simulink model "quad_new_leg_raibert_strategy_v5"  (R2022b)
settings: Solver=ode15s  StartTime=0.0  StopTime=5  RelTol=1e-3
undefined symbols (not defined in the file or in its folder): body, ctrl, ground, planner, X, Y, Z
libraries: nesl_utility x73, sm_lib x42, slpidlib x24, simulink x5, Contact_Forces_Lib x4, Parts_Lib x4, fl_lib x1, sharedtransform x1, dspstat3 x1
(part 5 of 5)

== system quad_new_leg_raibert_strategy_v5/leg_rr/u_joint_ctrl  ==
  tgt_angle : Inport
  has_ctrl : Inport  Port=2
  PID Controller : slpidlib/PID Controller  Controller=PID  Form=Parallel  TimeDomain=Continuous-time  UseExternalTs=off  SampleTime=-1  IntegratorMethod=Forward Euler  FilterMethod=Forward Euler  ControllerParametersSource=internal  P=ctrl.pos_kp  I=ctrl.pos_ki  UseKiTs=off  D=ctrl.pos_kd  N=100  UseFilter=on  TunerSelectOption=Transfer Function Based (PID Tuner App)  InitialConditionSource=internal  InitialConditionForIntegrator=0  InitialConditionForFilter=0  DifferentiatorICPrevScaledInput=0  ExternalReset=none  TrackingMode=off  Kt=1  LimitOutput=off  SatLimitsSource=internal  UpperSaturationLimit=inf  LowerSaturationLimit=-inf  LinearizeAsGain=on  AntiWindupMode=none  Kb=1  LimitIntegrator=off  UpperIntegratorSaturationLimit=inf  LowerIntegratorSaturationLimit=-inf  POutMin=[]  POutMax=[]  IOutMin=[]  IOutMax=[]  DOutMin=[]  DOutMax=[]  NOutMin=[]  NOutMax=[]  SumOutMin=[]  SumOutMax=[]  SaturationOutMin=[]  SaturationOutMax=[]  PParamMin=[]  PParamMax=[]  IParamMin=[]  IParamMax=[]  DParamMin=[]  DParamMax=[]  NParamMin=[]  NParamMax=[]  KbParamMin=[]  KbParamMax=[]  KtParamMin=[]  KtParamMax=[]  KbOutMin=[]  KbOutMax=[]  KtOutMin=[]  KtOutMax=[]  IntegratorOutMin=[]  IntegratorOutMax=[]  FilterOutMin=[]  FilterOutMax=[]  SumI1OutMin=[]  SumI1OutMax=[]  SumI2OutMin=[]  SumI2OutMax=[]  SumI3OutMin=[]  SumI3OutMax=[]  SumI4OutMin=[]  SumI4OutMax=[]  SumDOutMin=[]  SumDOutMax=[]  DifferentiatorOutMin=[]  DifferentiatorOutMax=[]  FilterDiffOutCoefMin=[]  FilterDiffOutCoefMax=[]  ReciprocalOutMin=[]  ReciprocalOutMax=[]  SumDenOutMin=[]  SumDenOutMax=[]  SumNumOutMin=[]  SumNumOutMax=[]  DivideOutMin=[]  DivideOutMax=[]  UdiffTsProdOutMin=[]  UdiffTsProdOutMax=[]  NTsProdOutMin=[]  NTsProdOutMax=[]  UintegralTsProdOutMin=[]  UintegralTsProdOutMax=[]  UngainTsProdOutMin=[]  UngainTsProdOutMax=[]  ClampingZeroOutDataTypeStr=Inherit: Inherit via back propagation  ClampingZeroOutMin=[]  ClampingZeroOutMax=[]  FilterDenConstantOutDataTypeStr=Inherit: Inherit via back propagation  FilterDenConstantOutMin=[]  FilterDenConstantOutMax=[]  PCopyOutDataTypeStr=Inherit: Inherit via back propagation  PCopyOutMin=[]  PCopyOutMax=[]  NCopyOutDataTypeStr=Inherit: Inherit via back propagation  NCopyOutMin=[]  NCopyOutMax=[]  IntegratorContinuousStateAttributes=''  IntegratorStateMustResolveToSignalObject=off  IntegratorRTWStateStorageClass=Auto  FilterContinuousStateAttributes=''  FilterStateMustResolveToSignalObject=off  FilterRTWStateStorageClass=Auto  ParallelPVariant=InternalParameters  IdealPVariant=Disabled  IVariant=InternalParameters  DVariant=InternalParameters  IntegratorVariant=Continuous  SatVariant=Disabled  AWVariant=Passthrough  PCopyVariant=Disabled  TRVariant=Disabled  FdbkBlocksVariant=Forward  IdealPFdbkVariant=Disabled  SatFdbkVariant=Disabled  DerivativeFilterVariant=ContFilter  NVariant=InternalParameters  NCopyVariant=Disabled  FilterICVariant=InternalICsFilter  IntegratorICVariant=InternalICs  ExternalResetVariant=Disabled  TRSumVariant=Passthrough  SumFdbkVariant=Disabled  SumVariant=Sum_PID  TsampFilterVariant=InternalTs  TsampNgainVariant=Passthrough  TsampIntegralVariant=Passthrough  ExternalSaturationOutDataTypeStr=Inherit: Same as second input
  PID Controller3 : slpidlib/PID Controller  Controller=PID  Form=Parallel  TimeDomain=Continuous-time  UseExternalTs=off  SampleTime=-1  IntegratorMethod=Forward Euler  FilterMethod=Forward Euler  ControllerParametersSource=internal  P=ctrl.vel_kp  I=ctrl.vel_ki  UseKiTs=off  D=ctrl.vel_kd  N=100  UseFilter=on  TunerSelectOption=Transfer Function Based (PID Tuner App)  InitialConditionSource=internal  InitialConditionForIntegrator=0  InitialConditionForFilter=0  DifferentiatorICPrevScaledInput=0  ExternalReset=none  TrackingMode=off  Kt=1  LimitOutput=off  SatLimitsSource=internal  UpperSaturationLimit=inf  LowerSaturationLimit=-inf  LinearizeAsGain=on  AntiWindupMode=none  Kb=1  LimitIntegrator=off  UpperIntegratorSaturationLimit=inf  LowerIntegratorSaturationLimit=-inf  POutMin=[]  POutMax=[]  IOutMin=[]  IOutMax=[]  DOutMin=[]  DOutMax=[]  NOutMin=[]  NOutMax=[]  SumOutMin=[]  SumOutMax=[]  SaturationOutMin=[]  SaturationOutMax=[]  PParamMin=[]  PParamMax=[]  IParamMin=[]  IParamMax=[]  DParamMin=[]  DParamMax=[]  NParamMin=[]  NParamMax=[]  KbParamMin=[]  KbParamMax=[]  KtParamMin=[]  KtParamMax=[]  KbOutMin=[]  KbOutMax=[]  KtOutMin=[]  KtOutMax=[]  IntegratorOutMin=[]  IntegratorOutMax=[]  FilterOutMin=[]  FilterOutMax=[]  SumI1OutMin=[]  SumI1OutMax=[]  SumI2OutMin=[]  SumI2OutMax=[]  SumI3OutMin=[]  SumI3OutMax=[]  SumI4OutMin=[]  SumI4OutMax=[]  SumDOutMin=[]  SumDOutMax=[]  DifferentiatorOutMin=[]  DifferentiatorOutMax=[]  FilterDiffOutCoefMin=[]  FilterDiffOutCoefMax=[]  ReciprocalOutMin=[]  ReciprocalOutMax=[]  SumDenOutMin=[]  SumDenOutMax=[]  SumNumOutMin=[]  SumNumOutMax=[]  DivideOutMin=[]  DivideOutMax=[]  UdiffTsProdOutMin=[]  UdiffTsProdOutMax=[]  NTsProdOutMin=[]  NTsProdOutMax=[]  UintegralTsProdOutMin=[]  UintegralTsProdOutMax=[]  UngainTsProdOutMin=[]  UngainTsProdOutMax=[]  ClampingZeroOutDataTypeStr=Inherit: Inherit via back propagation  ClampingZeroOutMin=[]  ClampingZeroOutMax=[]  FilterDenConstantOutDataTypeStr=Inherit: Inherit via back propagation  FilterDenConstantOutMin=[]  FilterDenConstantOutMax=[]  PCopyOutDataTypeStr=Inherit: Inherit via back propagation  PCopyOutMin=[]  PCopyOutMax=[]  NCopyOutDataTypeStr=Inherit: Inherit via back propagation  NCopyOutMin=[]  NCopyOutMax=[]  IntegratorContinuousStateAttributes=''  IntegratorStateMustResolveToSignalObject=off  IntegratorRTWStateStorageClass=Auto  FilterContinuousStateAttributes=''  FilterStateMustResolveToSignalObject=off  FilterRTWStateStorageClass=Auto  ParallelPVariant=InternalParameters  IdealPVariant=Disabled  IVariant=InternalParameters  DVariant=InternalParameters  IntegratorVariant=Continuous  SatVariant=Disabled  AWVariant=Passthrough  PCopyVariant=Disabled  TRVariant=Disabled  FdbkBlocksVariant=Forward  IdealPFdbkVariant=Disabled  SatFdbkVariant=Disabled  DerivativeFilterVariant=ContFilter  NVariant=InternalParameters  NCopyVariant=Disabled  FilterICVariant=InternalICsFilter  IntegratorICVariant=InternalICs  ExternalResetVariant=Disabled  TRSumVariant=Passthrough  SumFdbkVariant=Disabled  SumVariant=Sum_PID  TsampFilterVariant=InternalTs  TsampNgainVariant=Passthrough  TsampIntegralVariant=Passthrough  ExternalSaturationOutDataTypeStr=Inherit: Same as second input
  PSConv3 : nesl_utility/PS-Simulink Converter  PhysicalDomain=network_engine_domain  SubClassName=ps_output  LeftPortType=input  RightPortType=output  PseudoPeriodic=off  Frequencies=[]  VectorFormat=1-D array  Unit=1  AffineConversion=off
  PSConv4 : nesl_utility/PS-Simulink Converter  PhysicalDomain=network_engine_domain  SubClassName=ps_output  LeftPortType=input  RightPortType=output  PseudoPeriodic=off  Frequencies=[]  VectorFormat=1-D array  Unit=1  AffineConversion=off
  Product : Product
  SPConv : nesl_utility/Simulink-PS Converter  PhysicalDomain=network_engine_domain  SubClassName=ps_input  LeftPortType=input  RightPortType=output  PseudoPeriodic=off  Frequencies=[]  NoiseDistribution=none  NoiseParameters=[]  Unit=1  AffineConversion=off  FilteringAndDerivatives=filter  SimscapeFilterOrder=2  InputFilterTimeConstant=0.001  UdotUserProvided=1
  Sum1 : Sum  Inputs=|+-
  Sum6 : Sum  Inputs=|+-
  curr_angle : PMIOPort  Side=Left
  curr_omega : PMIOPort  Port=2  Side=Left
  torque : PMIOPort  Port=3  Side=Right
  wires:
  PSConv4/1 -> Sum6/2
  PID Controller3/1 -> Product/2
  has_ctrl/1 -> Product/1
  PSConv3/1 -> Sum1/2
  Product/1 -> SPConv/1
  Sum6/1 -> PID Controller3/1
  PID Controller/1 -> Sum6/1
  Sum1/1 -> PID Controller/1
  tgt_angle/1 -> Sum1/1
  connections:
  curr_omega/RConn1 -- PSConv4/LConn1
  SPConv/RConn1 -- torque/RConn1
  PSConv3/LConn1 -- curr_angle/RConn1

== matlab function quad_new_leg_raibert_strategy_v5/Controller/QuadCtrl ==
  settings: updateMethod=DISCRETE
  data: fl_ang input; tgt_ctrl_fl output; fr_ang input; rl_ang input; rr_ang input; contact_state input; body_R input; sensing_info input; tgt_ctrl_fr output; tgt_ctrl_rl output; tgt_ctrl_rr output; t input; body parameter; planner parameter; ctrl_state output; debug output
function [tgt_ctrl_fl,tgt_ctrl_fr,tgt_ctrl_rl,tgt_ctrl_rr, ctrl_state, debug] = ...
    controller(fl_ang, fr_ang, rl_ang, rr_ang, ...
    contact_state, body_R, sensing_info, t, body, planner)

% the sample time of the block is set to be 0.0025 (400Hz);
%walking code below is for it to turn right
%the left legs need to be stretched more in the x axis
dt = 0.0025;
%unpack sensing_info
body_vx = sensing_info(4);
body_vy = sensing_info(5);

fl_ang_s = fl_ang(1); fl_ang_u = fl_ang(2); fl_ang_k = fl_ang(3);
fr_ang_s = fr_ang(1); fr_ang_u = fr_ang(2); fr_ang_k = fr_ang(3);
rl_ang_s = rl_ang(1); rl_ang_u = rl_ang(2); rl_ang_k = rl_ang(3);
rr_ang_s = rr_ang(1); rr_ang_u = rr_ang(2); rr_ang_k = rr_ang(3);
% forward kinematics
fl_end_effector = forward_kinematics(fl_ang_s, fl_ang_u, fl_ang_k, body); 
rl_end_effector = forward_kinematics(rl_ang_s, rl_ang_u, rl_ang_k, body);
fr_end_effector = forward_kinematics(fr_ang_s, fr_ang_u, fr_ang_k, body);
rr_end_effector = forward_kinematics(rr_ang_s, rr_ang_u, rr_ang_k, body); 

% distance from center of mass to shoulder
fl_offset = [body.shoulder_distance;body.y_length/2+body.shoulder_size/2;0];
fr_offset = [body.shoulder_distance;-body.y_length/2-body.shoulder_size/2;0];
rl_offset = [-body.shoulder_distance;body.y_length/2+body.shoulder_size/2;0];
rr_offset = [-body.shoulder_distance;-body.y_length/2-body.shoulder_size/2;0];

%virtual leg1 fl (front left) rr(rear right) body frame
curr_virtual_leg1 = (fl_end_effector + fl_offset + rr_end_effector + rr_offset)*0.5;
%virtual leg2 fr (front right) rl(rear left) body frame 
curr_virtual_leg2 = (fr_end_effector + fr_offset + rl_end_effector + rl_offset)*0.5;


%decide state and state transition helpers
persistent state;
persistent timer;
persistent timer2;
persistent timer3;  % added extra time stopping (LIV)
persistent timer4;  % added extra time for right turn (LIV)

if isempty(state)
    state = 0;
end
if isempty(timer)
    timer = 0;
end
if isempty(timer2)
    timer2 = 0;
end
if isempty(timer3) %timer set to zero (LIV)
    timer3 = 0;
end
if isempty(timer4) %timer set to zero (LIV)
    timer4 = 0;
end

% init variables
           % fl fr rl rr
has_u_ctrl = [1 1 1 1];
normal_virtual_leg11 = [0;0;planner.stand_height];
normal_virtual_leg12 = [0;0;planner.stand_height];
normal_virtual_leg21 = [0;0;planner.stand_height];
normal_virtual_leg22 = [0;0;planner.stand_height];
move_fl_end_effector1 = normal_virtual_leg11;  %added by liv to split up leg
move_rr_end_effector1 = normal_virtual_leg12;
move_fr_end_effector1 = normal_virtual_leg21;
move_rl_end_effector1 = normal_virtual_leg22;

     
% state machine 

if state == 0 % standby state
    % in this state, just do nothing, but use time to make sure that all
    % feet stands on the ground 
    if contact_state(1) == 1 && contact_state(2) == 1 && contact_state(3) == 1 && contact_state(4) == 1
        %all foot on ground
        if abs(body_vx) < planner.state0_vel_thres 
            timer = timer + 1;
        else
            timer = 0;
        end
        if timer > planner.state0_trans_thres 
            state = 1;
            timer = 0;
        end
    end

elseif state == 1 % swing whole body to get a inital velocity
    timer2 = timer2 + 1;
    move_theta = planner.state0_swing_ang*sin(2*pi/planner.state0_swing_T*timer2);
    move_leg_Rx = [cos(move_theta) 0 sin(move_theta);
        0 1 0;
        -sin(move_theta) 0 cos(move_theta)];

    tgt_virtual_leg11_b = move_leg_Rx*normal_virtual_leg11;
    tgt_virtual_leg12_b = move_leg_Rx*normal_virtual_leg12;
    tgt_virtual_leg21_b = move_leg_Rx*normal_virtual_leg21;
    tgt_virtual_leg22_b = move_leg_Rx*normal_virtual_leg22;
    move_fl_end_effector1 = tgt_virtual_leg11_b;
    move_rr_end_effector1 = tgt_virtual_leg12_b;
    move_fr_end_effector1 = tgt_virtual_leg21_b;
    move_rl_end_effector1 = tgt_virtual_leg22_b;
        
    if body_vx > planner.state12_trans_speed
        timer = timer + 1;
    else
        timer = 0;
    end
    if timer > 40  %(keep a velocity larger than 0.2 for 0.1s)
        state = 2;
        timer = 0;
        timer2 = 0;
    end



elseif state == 2 %turn left on spot - FRONT LEFT (11)
    timer2 = timer2 + 1;

    if timer2 > planner.leg_swing_time %(0.5s finish movement)
        timer2 = planner.leg_swing_time;
    end

    has_u_ctrl = [1 0 0 0];
    t = timer2/planner.leg_swing_time;
    stance_length_coeff = 0.2*t^2 - 0.2*t + 1;
    tgt_virtual_leg11_b = stance_length_coeff*normal_virtual_leg11;
    move_fl_end_effector1 = tgt_virtual_leg11_b;
    length_coeff = 0.8*t^2-0.8*t+1;

    x_angle=-pi/15 %x needs to be negative to move forward
    move_leg_Rx = [cos(x_angle) 0 sin(x_angle);
        0 1 0;
        -sin(x_angle) 0 cos(x_angle)];
    tgt_virtual_leg11_b = length_coeff*move_leg_Rx*normal_virtual_leg11;

    y_angle=pi/15;  
    move_leg_Ry =[1 0 0;
                 0 cos(y_angle) -sin(y_angle);
                 0 sin(y_angle) cos(y_angle)];
    tgt_virtual_leg11_b = move_leg_Ry*tgt_virtual_leg11_b;

    move_fl_end_effector1 = body_R'*(tgt_virtual_leg11_b+fl_offset)-fl_offset;
    if norm(move_fl_end_effector1) > body.max_stretch
        move_fl_end_effector1 = move_fl_end_effector1/norm(move_fl_end_effector1)*body.max_stretch;
    end

   

    % state transition
    if timer2 > 0.5*planner.leg_swing_time && contact_state(2) == 1 && contact_state(3) == 1 && contact_state(4)
        timer = timer + 1;
    else
        timer = 0;
    end
    if timer > 10   % to be determined
        state = 3;
        timer = 0;
        timer2 = 0;
    end



elseif state == 3 %turn left on spot - REAR RIGHT (12)
    timer2 = timer2 + 1;

    if timer2 > planner.leg_swing_time %(0.5s finish movement)
        timer2 = planner.leg_swing_time;
    end

    has_u_ctrl = [0 0 0 1];
    t = timer2/planner.leg_swing_time;
    stance_length_coeff = 0.2*t^2 - 0.2*t + 1;
    tgt_virtual_leg12_b = stance_length_coeff*normal_virtual_leg12;
    move_rr_end_effector1 = tgt_virtual_leg12_b;
    length_coeff = 0.8*t^2-0.8*t+1;

    x_angle=-pi/15 %x needs to be negative to move forward
    move_leg_Rx = [cos(x_angle) 0 sin(x_angle);
        0 1 0;
        -sin(x_angle) 0 cos(x_angle)];
    tgt_virtual_leg12_b = length_coeff*move_leg_Rx*normal_virtual_leg12;

    y_angle=pi/20;  
    move_leg_Ry =[1 0 0;
                 0 cos(y_angle) -sin(y_angle);
                 0 sin(y_angle) cos(y_angle)];
    tgt_virtual_leg12_b = move_leg_Ry*tgt_virtual_leg12_b;

    move_rr_end_effector1 = body_R'*(tgt_virtual_leg12_b+rr_offset)-rr_offset;
    if norm(move_rr_end_effector1) > body.max_stretch
        move_rr_end_effector1 = move_rr_end_effector1/norm(move_rr_end_effector1)*body.max_stretch;
    end



      if timer2 > 0.5*planner.leg_swing_time && contact_state(2) == 1 && contact_state(3) == 1 && contact_state(4)
        timer = timer + 1;
    else
        timer = 0;
    end
    if timer > 10   % to be determined
        state = 4;
        timer = 0;
        timer2 = 0;
    end 



elseif state == 4 %turn left on spot - FRONT RIGHT (21)
    timer2 = timer2 + 1;

    if timer2 > planner.leg_swing_time %(0.5s finish movement)
        timer2 = planner.leg_swing_time;
    end

    has_u_ctrl = [0 1 0 0];
    t = timer2/planner.leg_swing_time;
    stance_length_coeff = 0.2*t^2 - 0.2*t + 1;
    tgt_virtual_leg21_b = stance_length_coeff*normal_virtual_leg21;
    move_fr_end_effector1 = tgt_virtual_leg21_b;
    length_coeff = 0.8*t^2-0.8*t+1;

    x_angle=-pi/15 %x needs to be negative to move forward
    move_leg_Rx = [cos(x_angle) 0 sin(x_angle);
        0 1 0;
        -sin(x_angle) 0 cos(x_angle)];
    tgt_virtual_leg21_b = length_coeff*move_leg_Rx*normal_virtual_leg21;

    y_angle=pi/20;  
    move_leg_Ry =[1 0 0;
                 0 cos(y_angle) -sin(y_angle);
                 0 sin(y_angle) cos(y_angle)];
    tgt_virtual_leg21_b = move_leg_Ry*tgt_virtual_leg21_b;

    move_fr_end_effector1 = body_R'*(tgt_virtual_leg21_b+fr_offset)-fr_offset;
    if norm(move_fr_end_effector1) > body.max_stretch
        move_fr_end_effector1 = move_fr_end_effector1/norm(move_fr_end_effector1)*body.max_stretch;
    end 


      if timer2 > 0.5*planner.leg_swing_time && contact_state(2) == 1 && contact_state(3) == 1 && contact_state(4)
        timer = timer + 1;
    else
        timer = 0;
    end
    if timer > 10   % to be determined
        state = 5;
        timer = 0;
        timer2 = 0;
    end 


elseif state == 5 %turn left on spot - REAR LEFT (22)
    timer2 = timer2 + 1;

    if timer2 > planner.leg_swing_time %(0.5s finish movement)
        timer2 = planner.leg_swing_time;
    end

    has_u_ctrl = [0 0 1 0];
    t = timer2/planner.leg_swing_time;
    stance_length_coeff = 0.2*t^2 - 0.2*t + 1;
    tgt_virtual_leg22_b = stance_length_coeff*normal_virtual_leg22;
    move_rl_end_effector1 = tgt_virtual_leg22_b;
    length_coeff = 0.8*t^2-0.8*t+1;

    x_angle=-pi/15 %x needs to be negative to move forward
    move_leg_Rx = [cos(x_angle) 0 sin(x_angle);
        0 1 0;
        -sin(x_angle) 0 cos(x_angle)];
    tgt_virtual_leg22_b = length_coeff*move_leg_Rx*normal_virtual_leg22;

    y_angle=pi/20;  
    move_leg_Ry =[1 0 0;
                 0 cos(y_angle) -sin(y_angle);
                 0 sin(y_angle) cos(y_angle)];
    tgt_virtual_leg22_b = move_leg_Ry*tgt_virtual_leg22_b;

    move_rl_end_effector1 = body_R'*(tgt_virtual_leg22_b+rl_offset)-rl_offset;
    if norm(move_rl_end_effector1) > body.max_stretch
        move_rl_end_effector1 = move_rl_end_effector1/norm(move_rl_end_effector1)*body.max_stretch;
    end 

end 

% elseif state == 2 % stance virtual leg1, swing virtual leg2 (fr-21 and rl-22)
%     timer2 = timer2 + 1;
%     if timer2 > planner.leg_swing_time %(0.5s finish movement)
%         timer2 = planner.leg_swing_time;
%     end
%     % stance leg no u control but need to balance the body
%                % fl fr rl rr
%     has_u_ctrl = [0 1 1 0];
%     t = timer2/planner.leg_swing_time;
% %     stance_length_coeff = 0.95+0.05*(timer2/planner.leg_swing_time);
%     stance_length_coeff = 0.2*t^2 - 0.2*t + 1;
%     tgt_virtual_leg11_b = stance_length_coeff*normal_virtual_leg11;  %code changed
%     tgt_virtual_leg12_b = stance_length_coeff*normal_virtual_leg12;
% 
%     move_fl_end_effector1 = tgt_virtual_leg11_b; %Code changed
%     move_rr_end_effector1 = tgt_virtual_leg12_b;
%     
%     
%     % swing leg must consider body angle 
% %     move_theta = -11/180*pi*(t);
%     length_coeff = 0.8*t^2-0.8*t+1;
% 
%     % MOVE LEG IN X DIRECTION
%     %front right leg - 21
%     move_theta = get_move_angle(length_coeff*normal_virtual_leg21,body_vx, planner.tgt_body_vx, planner);
%     move_leg_Rx = [cos(move_theta) 0 sin(move_theta);
%         0 1 0;
%         -sin(move_theta) 0 cos(move_theta)];
%     tgt_virtual_leg21_b = length_coeff*move_leg_Rx*normal_virtual_leg21;
% 
%     %rear left - 22
%     move_theta = get_move_angle1(length_coeff*normal_virtual_leg22,body_vx, planner.tgt_body_vx, planner);
%     move_leg_Rx = [cos(move_theta) 0 sin(move_theta);
%         0 1 0;
%         -sin(move_theta) 0 cos(move_theta)];
%     tgt_virtual_leg22_b = length_coeff*move_leg_Rx*normal_virtual_leg22;
% 
% 
% 
%     % MOVE LEG IN Y DIRECTION
%     %front right leg - 21
%     sagittal_angle = get_sagittal_angle(tgt_virtual_leg21_b,body_R, body_vy, planner);
%     move_leg_Ry =[1 0 0;
%                  0 cos(sagittal_angle) -sin(sagittal_angle);
%                  0 sin(sagittal_angle) cos(sagittal_angle)];
%     tgt_virtual_leg21_b = move_leg_Ry*tgt_virtual_leg21_b;
% 
%     %Rear left leg - 22
%     sagittal_angle = get_sagittal_angle(tgt_virtual_leg22_b,body_R, body_vy, planner);
%     move_leg_Ry =[1 0 0;
%                  0 cos(sagittal_angle) -sin(sagittal_angle);
%                  0 sin(sagittal_angle) cos(sagittal_angle)];
%     tgt_virtual_leg22_b = move_leg_Ry*tgt_virtual_leg22_b;
% 
% 
%     
%     %MOVE LEG IN Z DIRECTION ADDED by LIV
%     %front right leg - 21
%        z_angle = pi/3;
%        move_leg_Rz=[cos(z_angle) -sin(z_angle) 0;
%                     sin(z_angle) cos(z_angle),0;
%                     0                0         1];
%        tgt_virtual_leg21_b = move_leg_Rz*tgt_virtual_leg21_b;
% 
%      %rear left leg - 22
%        z_angle = pi/3;
%        move_leg_Rz=[cos(z_angle) -sin(z_angle) 0;
%                     sin(z_angle) cos(z_angle),0;
%                     0                0         1];
%        tgt_virtual_leg22_b = move_leg_Rz*tgt_virtual_leg22_b;
%   
% 
%     
%     
%     move_fr_end_effector1 = body_R'*(tgt_virtual_leg21_b+fr_offset)-fr_offset;
%     if norm(move_fr_end_effector1) > body.max_stretch
%         move_fr_end_effector1 = move_fr_end_effector1/norm(move_fr_end_effector1)*body.max_stretch;
%     end
%     move_rl_end_effector1 = body_R'*(tgt_virtual_leg22_b+rl_offset)-rl_offset;
%     if norm(move_rl_end_effector1) > body.max_stretch
%         move_rl_end_effector1 = move_rl_end_effector1/norm(move_rl_end_effector1)*body.max_stretch;
%     end
% end

%     
%     % state transition
% %     if timer2 == planner.leg_swing_time
%     if timer2 > 0.5*planner.leg_swing_time && contact_state(2) == 1 && contact_state(3) == 1
%         timer = timer + 1;
%     else
%         timer = 0;
%     end
%     if timer > 10   % to be determined
%         state = 3;
%         timer = 0;
%         timer2 = 0;
%     end
%   
% 
% 
% elseif state == 3 % swing virtual leg1 (fl-11 and rr-12), stance virtual leg2
%     timer2 = timer2 + 1;
%     if timer2 > planner.leg_swing_time %(0.5s finish movement)
%         timer2 = planner.leg_swing_time;
%     end
%     % stance leg no u control but need to balance the body
%                % fl fr rl rr
%     has_u_ctrl = [1 0 0 1];
% %     stance_length_coeff = 0.95+0.05*(timer2/planner.leg_swing_time);
%     t = timer2/planner.leg_swing_time;
%     stance_length_coeff = 0.2*t^2 - 0.2*t + 1;
%     tgt_virtual_leg21_b = stance_length_coeff*normal_virtual_leg21;
%     tgt_virtual_leg22_b = stance_length_coeff*normal_virtual_leg22;
% 
%     move_fr_end_effector = tgt_virtual_leg21_b;
%     move_rl_end_effector = tgt_virtual_leg22_b;
%     
%     % swing leg must consider body angle 
%     % theta is a function of forward velocity 
% %     move_theta = -11/180*pi*(t);
%     length_coeff = 0.8*t^2-0.8*t+1;
%     %tgt_virtual_leg2_b = length_coeff*eye(3)*normal_virtual_leg2; %added by LIV
% 
%         % MOVE LEG IN X DIRECTION
%         %front left leg
%     move_theta = get_move_angle1(length_coeff*normal_virtual_leg11,body_vx, planner.tgt_body_vx, planner);
%     move_leg_Rx = [cos(move_theta) 0 sin(move_theta);
%         0 1 0;
%         -sin(move_theta) 0 cos(move_theta)];
%     tgt_virtual_leg11_b = length_coeff*move_leg_Rx*normal_virtual_leg11;
% 
%        %rear right leg
%     move_theta = get_move_angle(length_coeff*normal_virtual_leg12,body_vx, planner.tgt_body_vx, planner);
%     move_leg_Rx = [cos(move_theta) 0 sin(move_theta);
%         0 1 0;
%         -sin(move_theta) 0 cos(move_theta)];
%     tgt_virtual_leg12_b = length_coeff*move_leg_Rx*normal_virtual_leg12;
% 
%         % MOVE LEG IN Y DIRECTION
%         %front left leg
%     sagittal_angle = get_sagittal_angle(tgt_virtual_leg11_b,body_R, body_vy, planner);
%     move_leg_Ry =[1 0 0;
%                  0 cos(sagittal_angle) -sin(sagittal_angle);
%                  0 sin(sagittal_angle) cos(sagittal_angle)];
%     tgt_virtual_leg11_b = move_leg_Ry*tgt_virtual_leg11_b;
% 
%         %rear right leg
%     sagittal_angle = get_sagittal_angle(tgt_virtual_leg12_b,body_R, body_vy, planner);
%     move_leg_Ry =[1 0 0;
%                  0 cos(sagittal_angle) -sin(sagittal_angle);
%                  0 sin(sagittal_angle) cos(sagittal_angle)];
%     tgt_virtual_leg12_b = move_leg_Ry*tgt_virtual_leg12_b;
% 
% 
%        %MOVE LEG IN Z DIRECTION ADDED by LIV
%        %front left leg
%        z_angle= pi/3;
%        move_leg_Rz=[cos(z_angle) -sin(z_angle) 0;
%                     sin(z_angle) cos(z_angle),0;
%                     0                0         1];
%        tgt_virtual_leg11_b = move_leg_Rz*tgt_virtual_leg11_b;   %is this virtual leg 1 or 2, i changed to 1 from 2
% 
%        %rear right leg
%        z_angle=pi/3;
%        move_leg_Rz=[cos(z_angle) -sin(z_angle) 0;
%                     sin(z_angle) cos(z_angle),0;
%                     0                0         1];
%        tgt_virtual_leg12_b = move_leg_Rz*tgt_virtual_leg12_b;
% 
%     
%     move_fl_end_effector1 = body_R'*(tgt_virtual_leg11_b+fl_offset)-fl_offset;
%     if norm(move_fl_end_effector1) > body.max_stretch
%         move_fl_end_effector1 = move_fl_end_effector1/norm(move_fl_end_effector1)*body.max_stretch;
%     end
%     move_rr_end_effector1 = body_R'*(tgt_virtual_leg12_b+rr_offset)-rr_offset;
%     if norm(move_rr_end_effector1) > body.max_stretch
%         move_rr_end_effector1 = move_rr_end_effector1/norm(move_rr_end_effector1)*body.max_stretch;
%     end
%     
%     % state transition
%     % if timer2 == planner.leg_swing_time
%     if timer2 > 0.5*planner.leg_swing_time && contact_state(1) == 1 && contact_state(4) == 1  
%         timer = timer + 1;
%     else
%         timer = 0;
%     end
%     if timer > 2   % to be determined
%         state = 2;
%         timer = 0; 
%         timer2 = 0;
%     end
%     if  timer > 4
%             state = 4;
%             timer = 0;
%             timer2 = 0;
%             timer3 = 0;
%     end


%new states added by LIV 
% elseif state == 4 % STOPPING of body (LIV)
%     timer3 = timer3 + 1;    
%       if timer3 > planner.leg_swing_time %(0.5s finish movement)
%         timer3 = planner.leg_swing_time;
%       end
%  if contact_state(1) == 1 && contact_state(2) == 1 && contact_state(3) == 1 && contact_state(4) == 1
%         %all foot on ground
%         if abs(body_vx) < planner.state0_vel_thres 
%             timer3 = timer3 + 1;
%         else
%             timer3 = 0;
%         end
%         if timer3 > planner.state0_trans_thres 
%             state = 5;
%             timer3 = 0;
%         end
%         
%  end 
% 
% 
% %new state added by LIV
% elseif state == 5 %rotation to RIGHT (Liv)
%     timer4 = timer4 + 1;



%  end



%% fl to joint
[inv_s,inv_u,inv_k] = inverse_kinematics(move_fl_end_effector1, body);
fl_tgt_ang_s = inv_s; 
fl_tgt_ang_u = inv_u;       
fl_tgt_ang_k = inv_k; 
tgt_ctrl_fl = [fl_tgt_ang_s;fl_tgt_ang_u;fl_tgt_ang_k;has_u_ctrl(1)];

%% fr to joint
[inv_s,inv_u,inv_k] = inverse_kinematics(move_fr_end_effector1, body);
fr_tgt_ang_s = inv_s;
fr_tgt_ang_u = inv_u;
fr_tgt_ang_k = inv_k;
tgt_ctrl_fr = [fr_tgt_ang_s;fr_tgt_ang_u;fr_tgt_ang_k;has_u_ctrl(2)];

%% rl to joint
[inv_s,inv_u,inv_k] = inverse_kinematics(move_rl_end_effector1, body);
rl_tgt_ang_s = inv_s;
rl_tgt_ang_u = inv_u;
rl_tgt_ang_k = inv_k;
tgt_ctrl_rl = [rl_tgt_ang_s;rl_tgt_ang_u;rl_tgt_ang_k;has_u_ctrl(3)];

%% rr to joint
[inv_s,inv_u,inv_k] = inverse_kinematics(move_rr_end_effector1, body);
rr_tgt_ang_s = inv_s;
rr_tgt_ang_u = inv_u;
rr_tgt_ang_k = inv_k; 
tgt_ctrl_rr = [rr_tgt_ang_s;rr_tgt_ang_u;rr_tgt_ang_k;has_u_ctrl(4)];

ctrl_state = state;
debug = timer;

end


%new function based off below two functions for z plane movement
%created by LIV
function move_angle = get_z_angle(virtual_leg, body_vz, planner)

    distance = body_vz* planner.z_Ts/2 + planner.z_Kv*(0-body_vz);  

    if distance > 0.5*norm(virtual_leg)
        distance = 0.5*norm(virtual_leg);
    elseif distance < -0.5*norm(virtual_leg)
        distance = -0.5*norm(virtual_leg);
    end
    
    move_angle = asin(distance/norm(virtual_leg));
    if move_angle > 20/180*pi
        move_angle = 20/180*pi;
    elseif move_angle < -20/180*pi
        move_angle = -20/180*pi;
    end
    
end



% original function
function move_angle = get_move_angle(virtual_leg,body_vx, tgt_body_vx, planner)

    distance = body_vx* planner.Ts/2 + planner.Kv*(tgt_body_vx-body_vx);
    
    if distance > 0.5*norm(virtual_leg)
        distance = 0.5*norm(virtual_leg);
    elseif distance < -0.5*norm(virtual_leg)
        distance = -0.5*norm(virtual_leg);
    end
    
    move_angle = asin(distance/norm(virtual_leg));
    if move_angle > 20/180*pi
        move_angle = 20/180*pi;      
    elseif move_angle < -20/180*pi
        move_angle = -20/180*pi;
    end
    
end


% function copied from above and changed
function move_angle1 = get_move_angle1(virtual_leg,body_vx, tgt_body_vx, planner)

    distance = body_vx* planner.Ts/2 + planner.Kv*(tgt_body_vx-body_vx);
    
    if distance > 0.5*norm(virtual_leg)
        distance = 0.5*norm(virtual_leg);
    elseif distance < -0.5*norm(virtual_leg)
        distance = -0.5*norm(virtual_leg);
    end
    
    move_angle1 = asin(distance/norm(virtual_leg));
    if move_angle1 > 20/180*pi
        move_angle1 = 20/180*pi;      %code changed from 20 to 75
    elseif move_angle1 < -20/180*pi
        move_angle1 = -20/180*pi;
    end
    
end

function move_angle = get_sagittal_angle(virtual_leg, body_R, body_vy, planner)

    distance = body_vy* planner.y_Ts/2 + planner.y_Kv*(0-body_vy);  

    if distance > 0.5*norm(virtual_leg)
        distance = 0.5*norm(virtual_leg);
    elseif distance < -0.5*norm(virtual_leg)
        distance = -0.5*norm(virtual_leg);
    end
    
    move_angle = asin(distance/norm(virtual_leg));
    if move_angle > 20/180*pi
        move_angle = 20/180*pi;
    elseif move_angle < -20/180*pi
        move_angle = -20/180*pi;
    end
    
end
